simulink model "Desc_model"  (R2017a)
settings: Solver=VariableStepAuto  StartTime=0.0  StopTime=9.9  RelTol=1e-3
values from neighbouring files (symbols this model uses):
  A = double(subs(A_sym, phi_sym, 0))    [create_constants.m]    (also in forward_kinematic_linear.m = [0.7689, 0.0639, -0.1471, 0.0592; linearize_model.m = -1*((Rt / k_m * Z)\(Rt / k_m * V + EM * eye(4,4))); sim_system.m; test.m = [cos(phi), -sin(phi), 0)
  B = double(subs(B_sym, phi_sym, 0))    [create_constants.m]    (also in forward_kinematic_linear.m = [6.8984, -1.9066, 4.3907, -1.7678; linearize_model.m = pinv(Rt / k_m * Z); sim_system.m; test.m = [m, 0, 0)
  BotToWheel = G' / r    [create_constants.m]    (also in find_body_to_wheel_alpha.m = (-1 * G / r)'; graph_max_robot_speeds.m; sim_system.m; test_kalman_filter_LQI.m = -1 * G' / r)
  C = eye(4,4)    [create_constants.m]    (also in sim_system.m; test.m = simplify(C); test_kalman_filter_LQI.m; test_kalman_filter_LQR.m)
  camera_ts = 0.01    [create_constants.m]
  D = zeros(4,4)    [create_constants.m]    (also in sim_system.m; test.m = pinv(G); test_kalman_filter_LQI.m; test_kalman_filter_LQR.m)
  delay_sample = 0    [create_constants.m]
  encoder_ts = 0.01    [create_constants.m]
  td = 0    [create_constants.m]    (also in sim_system.m)
  ti = 0    [create_constants.m]    (also in sim_system.m)
  tp = 0    [create_constants.m]    (also in sim_system.m = 2)
  wd = 0    [create_constants.m]    (also in sim_system.m)
  WheelToBot = pinv(BotToWheel)    [create_constants.m]    (also in graph_max_robot_speeds.m; sim_system.m; test_kalman_filter_LQI.m; test_kalman_filter_LQR.m)
  wi = 0    [create_constants.m]    (also in sim_system.m = 0.5)
  wp = 0    [create_constants.m]    (also in sim_system.m = 1)
  X_0 = [0, 0, 0, 0]    [create_constants.m]
undefined symbols (not defined in the file or in its folder): K_int
libraries: simulink x4
settings Model: Creator=Joe  LastModifiedBy=Joe

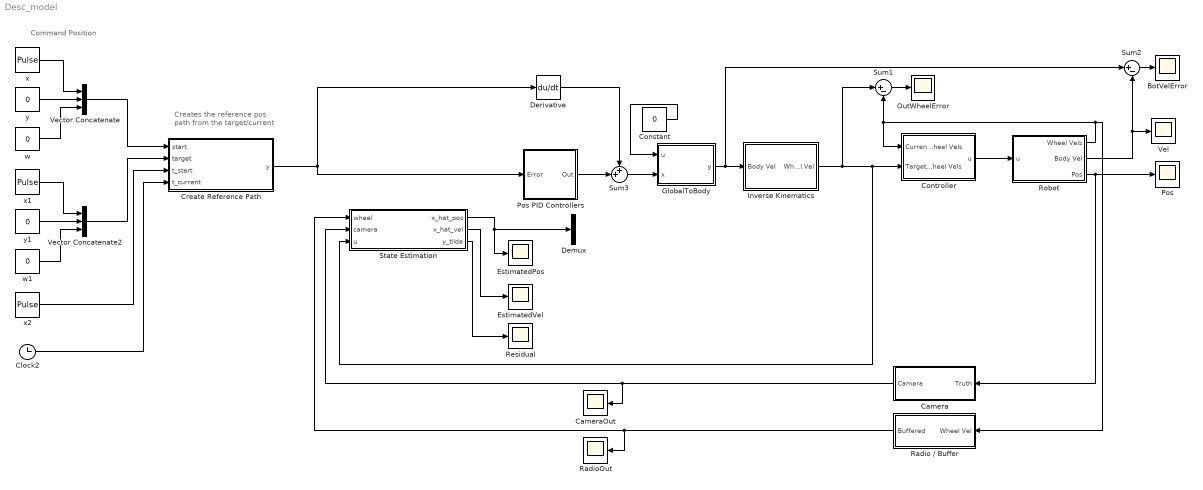
== system Desc_model ==
  note: Command Position
  note: Creates the reference pos
      | path from the target/current
  BotVelError : Scope
  Camera : Subsystem
  CameraOut : Scope
  Clock2 : Clock
  Constant : Constant  Value=0
  Controller : Subsystem
  Create Reference Path : MATLAB Function  TreatAsAtomicUnit=on
  Demux : Demux  Outputs=3
  Derivative : Derivative
  EstimatedPos : Scope
  EstimatedVel : Scope
  GlobalToBody : MATLAB Function  TreatAsAtomicUnit=on
  Inverse Kinematics : Subsystem
  OutWheelError : Scope
  Pos : Scope
  Pos PID Controllers : Subsystem
  Radio / Buffer : Subsystem
  RadioOut : Scope
  Residual : Scope
  Robot : Subsystem
  State Estimation : MATLAB Function  TreatAsAtomicUnit=on
  Sum1 : Sum  Inputs=|+-
  Sum2 : Sum  Inputs=|+-
  Sum3 : Sum  Inputs=++|
  Vector Concatenate : Concatenate  NumInputs=3
  Vector Concatenate2 : Concatenate  NumInputs=3
  Vel : Scope
  w : Constant  Value=0
  w1 : Constant  Value=0
  x : DiscretePulseGenerator  PulseType=Time based  Period=10  PulseWidth=50  PhaseDelay=5
  x1 : DiscretePulseGenerator  PulseType=Time based  Period=10  PulseWidth=50
  x2 : DiscretePulseGenerator  PulseType=Time based  Amplitude=5  Period=20  PulseWidth=50  PhaseDelay=5
  y : Constant  Value=0
  y1 : Constant  Value=0
  wires:
  Sum1/1 -> OutWheelError/1
  Sum2/1 -> BotVelError/1
  GlobalToBody/1(y) -> Sum2/1, Inverse Kinematics/1(Body Vel)
  Robot/1(Wheel Vels) -> Radio / Buffer/1(Wheel Vel), Controller/1(Current Wheel Vels), Sum1/2
  Controller/1(u) -> Robot/1(u)
  Inverse Kinematics/1(Wheel Vel) -> State Estimation/3(u), Controller/2(Target Wheel Vels), Sum1/1
  Robot/2(Body Vel) -> Vel/1, Sum2/2
  Robot/3(Pos) -> Camera/1(Truth), Pos/1
  w/1 -> Vector Concatenate/3
  Clock2/1 -> Create Reference Path/4(t_current)
  y/1 -> Vector Concatenate/2
  x1/1 -> Vector Concatenate2/1
  y1/1 -> Vector Concatenate2/2
  w1/1 -> Vector Concatenate2/3
  Vector Concatenate2/1 -> Create Reference Path/2(target)
  Vector Concatenate/1 -> Create Reference Path/1(start)
  x/1 -> Vector Concatenate/1
  x2/1 -> Create Reference Path/3(t_start)
  Camera/1(Camera) -> CameraOut/1, State Estimation/2(camera)
  Radio / Buffer/1(Buffered) -> RadioOut/1, State Estimation/1(wheel)
  State Estimation/1(x_hat_pos) -> Demux/1, EstimatedPos/1
  Sum3/1 -> GlobalToBody/2(x)
  Derivative/1 -> Sum3/1
  Pos PID Controllers/1(Out) -> Sum3/2
  State Estimation/3(y_tilda) -> Residual/1
  State Estimation/2(x_hat_vel) -> EstimatedVel/1
  Create Reference Path/1(y) -> Pos PID Controllers/1(Error), Derivative/1
  Constant/1 -> GlobalToBody/1(u)

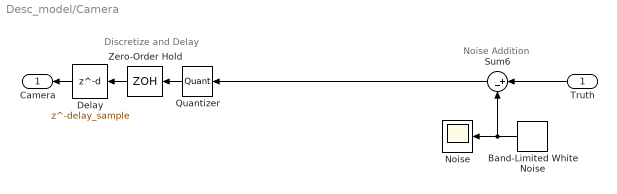
== system Desc_model/Camera ==
  note: Noise Addition
  note: Discretize and Delay
  Truth : Inport
  Band-Limited White Noise : simulink/Sources/Band-Limited White Noise  Cov=camera_noise  Ts=camera_ts  seed=[23341]
  Delay : Delay  DelayLength=delay_sample
  Noise : Scope
  Quantizer : Quantizer  QuantizationInterval=0.01
  Sum6 : Sum  Inputs=|+-
  Zero-Order Hold : ZeroOrderHold  SampleTime=camera_ts
  Camera : Outport
  wires:
  Delay/1 -> Camera/1
  Truth/1 -> Sum6/1
  Band-Limited White Noise/1 -> Noise/1, Sum6/2
  Quantizer/1 -> Zero-Order Hold/1
  Zero-Order Hold/1 -> Delay/1
  Sum6/1 -> Quantizer/1

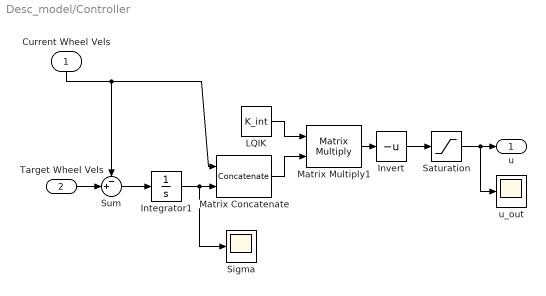
== system Desc_model/Controller ==
  Current Wheel Vels : Inport
  Target Wheel Vels : Inport  Port=2
  Integrator1 : Integrator
  Invert : UnaryMinus
  LQIK : Constant  Value=K_int
  Matrix Concatenate : Concatenate
  Matrix Multiply1 : Product  Multiplication=Matrix(*)
  Saturation : Saturate  UpperLimit=12  LowerLimit=-12
  Sigma : Scope
  Sum : Sum  Inputs=-+|
  u_out : Scope
  u : Outport
  wires:
  Invert/1 -> Saturation/1
  Integrator1/1 -> Sigma/1, Matrix Concatenate/2
  Sum/1 -> Integrator1/1
  Matrix Multiply1/1 -> Invert/1
  LQIK/1 -> Matrix Multiply1/1
  Matrix Concatenate/1 -> Matrix Multiply1/2
  Current Wheel Vels/1 -> Matrix Concatenate/1, Sum/1
  Target Wheel Vels/1 -> Sum/2
  Saturation/1 -> u_out/1, u/1

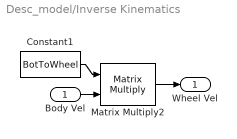
== system Desc_model/Inverse Kinematics ==
  Body Vel : Inport
  Constant1 : Constant  Value=BotToWheel
  Matrix Multiply2 : Product  Multiplication=Matrix(*)
  Wheel Vel : Outport
  wires:
  Constant1/1 -> Matrix Multiply2/1
  Body Vel/1 -> Matrix Multiply2/2
  Matrix Multiply2/1 -> Wheel Vel/1

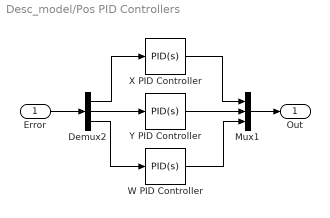
== system Desc_model/Pos PID Controllers ==
  Error : Inport
  Demux2 : Demux  Outputs=3
  Mux1 : Mux  Inputs=3
  W PID Controller : simulink/Continuous/PID Controller  Controller=PID  TimeDomain=Continuous-time  SampleTime=-1  IntegratorMethod=Forward Euler  FilterMethod=Forward Euler  Form=Parallel  UseFilter=on  ControllerParametersSource=internal  P=wp  I=wi  D=wd  N=26080.4758865559  InitialConditionSource=internal  InitialConditionForIntegrator=0  InitialConditionForFilter=0  ExternalReset=none  LimitOutput=off  UpperSaturationLimit=inf  LowerSaturationLimit=-inf  LinearizeAsGain=on  AntiWindupMode=none  Kb=1  TrackingMode=off  Kt=1  PParamMin=[]  PParamMax=[]  IParamMin=[]  IParamMax=[]  DParamMin=[]  DParamMax=[]  NParamMin=[]  NParamMax=[]  KbParamMin=[]  KbParamMax=[]  KtParamMin=[]  KtParamMax=[]  POutMin=[]  POutMax=[]  IOutMin=[]  IOutMax=[]  DOutMin=[]  DOutMax=[]  NOutMin=[]  NOutMax=[]  KbOutMin=[]  KbOutMax=[]  KtOutMin=[]  KtOutMax=[]  IntegratorOutMin=[]  IntegratorOutMax=[]  FilterOutMin=[]  FilterOutMax=[]  SumOutMin=[]  SumOutMax=[]  SumI1OutMin=[]  SumI1OutMax=[]  SumI2OutMin=[]  SumI2OutMax=[]  SumI3OutMin=[]  SumI3OutMax=[]  SumDOutMin=[]  SumDOutMax=[]  SaturationOutMin=[]  SaturationOutMax=[]  IntegratorContinuousStateAttributes=''  IntegratorStateMustResolveToSignalObject=off  IntegratorRTWStateStorageClass=Auto  FilterContinuousStateAttributes=''  FilterStateMustResolveToSignalObject=off  FilterRTWStateStorageClass=Auto  DifferentiatorICPrevScaledInput=0  DifferentiatorOutMin=[]  DifferentiatorOutMax=[]  InitialConditionSetting=State (most efficient)
  X PID Controller : simulink/Continuous/PID Controller  Controller=PID  TimeDomain=Continuous-time  SampleTime=-1  IntegratorMethod=Forward Euler  FilterMethod=Forward Euler  Form=Parallel  UseFilter=on  ControllerParametersSource=internal  P=tp  I=ti  D=td  N=0  InitialConditionSource=internal  InitialConditionForIntegrator=0  InitialConditionForFilter=0  ExternalReset=none  LimitOutput=off  UpperSaturationLimit=inf  LowerSaturationLimit=-inf  LinearizeAsGain=on  AntiWindupMode=none  Kb=1  TrackingMode=off  Kt=1  PParamMin=[]  PParamMax=[]  IParamMin=[]  IParamMax=[]  DParamMin=[]  DParamMax=[]  NParamMin=[]  NParamMax=[]  KbParamMin=[]  KbParamMax=[]  KtParamMin=[]  KtParamMax=[]  POutMin=[]  POutMax=[]  IOutMin=[]  IOutMax=[]  DOutMin=[]  DOutMax=[]  NOutMin=[]  NOutMax=[]  KbOutMin=[]  KbOutMax=[]  KtOutMin=[]  KtOutMax=[]  IntegratorOutMin=[]  IntegratorOutMax=[]  FilterOutMin=[]  FilterOutMax=[]  SumOutMin=[]  SumOutMax=[]  SumI1OutMin=[]  SumI1OutMax=[]  SumI2OutMin=[]  SumI2OutMax=[]  SumI3OutMin=[]  SumI3OutMax=[]  SumDOutMin=[]  SumDOutMax=[]  SaturationOutMin=[]  SaturationOutMax=[]  IntegratorContinuousStateAttributes=''  IntegratorStateMustResolveToSignalObject=off  IntegratorRTWStateStorageClass=Auto  FilterContinuousStateAttributes=''  FilterStateMustResolveToSignalObject=off  FilterRTWStateStorageClass=Auto  DifferentiatorICPrevScaledInput=0  DifferentiatorOutMin=[]  DifferentiatorOutMax=[]  InitialConditionSetting=State (most efficient)
  Y PID Controller : simulink/Continuous/PID Controller  Controller=PID  TimeDomain=Continuous-time  SampleTime=-1  IntegratorMethod=Forward Euler  FilterMethod=Forward Euler  Form=Parallel  UseFilter=on  ControllerParametersSource=internal  P=tp  I=ti  D=td  N=0  InitialConditionSource=internal  InitialConditionForIntegrator=0  InitialConditionForFilter=0  ExternalReset=none  LimitOutput=off  UpperSaturationLimit=inf  LowerSaturationLimit=-inf  LinearizeAsGain=on  AntiWindupMode=none  Kb=1  TrackingMode=off  Kt=1  PParamMin=[]  PParamMax=[]  IParamMin=[]  IParamMax=[]  DParamMin=[]  DParamMax=[]  NParamMin=[]  NParamMax=[]  KbParamMin=[]  KbParamMax=[]  KtParamMin=[]  KtParamMax=[]  POutMin=[]  POutMax=[]  IOutMin=[]  IOutMax=[]  DOutMin=[]  DOutMax=[]  NOutMin=[]  NOutMax=[]  KbOutMin=[]  KbOutMax=[]  KtOutMin=[]  KtOutMax=[]  IntegratorOutMin=[]  IntegratorOutMax=[]  FilterOutMin=[]  FilterOutMax=[]  SumOutMin=[]  SumOutMax=[]  SumI1OutMin=[]  SumI1OutMax=[]  SumI2OutMin=[]  SumI2OutMax=[]  SumI3OutMin=[]  SumI3OutMax=[]  SumDOutMin=[]  SumDOutMax=[]  SaturationOutMin=[]  SaturationOutMax=[]  IntegratorContinuousStateAttributes=''  IntegratorStateMustResolveToSignalObject=off  IntegratorRTWStateStorageClass=Auto  FilterContinuousStateAttributes=''  FilterStateMustResolveToSignalObject=off  FilterRTWStateStorageClass=Auto  DifferentiatorICPrevScaledInput=0  DifferentiatorOutMin=[]  DifferentiatorOutMax=[]  InitialConditionSetting=State (most efficient)
  Out : Outport
  wires:
  Error/1 -> Demux2/1
  Mux1/1 -> Out/1
  X PID Controller/1 -> Mux1/1
  Demux2/2 -> Y PID Controller/1
  W PID Controller/1 -> Mux1/3
  Demux2/1 -> X PID Controller/1
  Y PID Controller/1 -> Mux1/2
  Demux2/3 -> W PID Controller/1

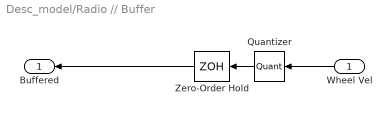
== system Desc_model/Radio // Buffer ==
  Wheel Vel : Inport
  Quantizer : Quantizer  QuantizationInterval=0.01
  Zero-Order Hold : ZeroOrderHold  SampleTime=encoder_ts
  Buffered : Outport
  wires:
  Zero-Order Hold/1 -> Buffered/1
  Wheel Vel/1 -> Quantizer/1
  Quantizer/1 -> Zero-Order Hold/1

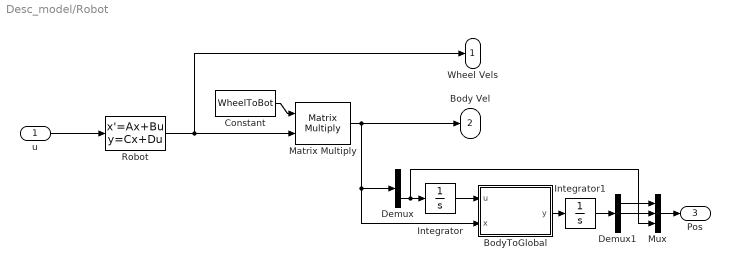
== system Desc_model/Robot ==
  u : Inport
  BodyToGlobal : MATLAB Function  TreatAsAtomicUnit=on
  Constant : Constant  Value=WheelToBot
  Demux : Demux  Outputs=3
  Demux1 : Demux  Outputs=3
  Integrator : Integrator
  Integrator1 : Integrator
  Matrix Multiply : Product  Multiplication=Matrix(*)
  Mux : Mux  Inputs=3
  Robot : StateSpace  A=A  B=B  C=C  D=D  X0=X_0
  Wheel Vels : Outport
  Body Vel : Outport  Port=2
  Pos : Outport  Port=3
  wires:
  Robot/1 -> Wheel Vels/1, Matrix Multiply/2
  Matrix Multiply/1 -> BodyToGlobal/2(x), Demux/1, Body Vel/1
  Constant/1 -> Matrix Multiply/1
  u/1 -> Robot/1
  Demux/3 -> Mux/3, Integrator/1
  Integrator/1 -> BodyToGlobal/1(u)
  Demux1/2 -> Mux/2
  Demux1/1 -> Mux/1
  Mux/1 -> Pos/1
  BodyToGlobal/1(y) -> Integrator1/1
  Integrator1/1 -> Demux1/1

== matlab function Desc_model/Create Reference Path ==
  data: start input; target input; y output; t_start input; t_current input
function y = Create_Ref(start, target, t_start, t_current)
y = zeros(3,1);
for i = 1:3
    a_c = 2; % Max Accel
    s_c = 1; % Max Speed
    t_a = s_c / a_c;
    
    sign = 2*(target(i) > start(i)) - 1;
    
    t_s = sign*(target(i) - start(i))/s_c - t_a;
    t_end = t_start + t_a + t_s + t_a;

    if (abs(start(i) - target(i)) < 0.01)
        y(i) = 0;
        continue;
    end
    
    if t_current < t_start
        y(i) = start(i);
    elseif t_current < t_start + t_a
        y(i) = start(i) + sign*1/2*a_c*(t_current - t_start)^2;
    elseif t_current < t_end - t_a
        y(i) = 1/2*(start(i) + target(i)) + sign*s_c*(t_current - 1/2*(t_start + t_end));
    elseif t_current < t_end
        y(i) = target(i) - sign*1/2*a_c*(t_end - t_current)^2;
    else % t_current > t_end
        y(i) = target(i);
    end
end

== matlab function Desc_model/Robot/BodyToGlobal ==
  data: u input; y output; x input
function y =  rotate(u, x)

r = [cos(u), -sin(u), 0;
     sin(u),  cos(u), 0;
          0,       0, 1];
y = r*x;

== matlab function Desc_model/GlobalToBody ==
  data: u input; y output; x input
function y =  rotate(u, x)

r = [cos(u), -sin(u), 0;
     sin(u),  cos(u), 0;
          0,       0, 1];
y = r*x;

== matlab function Desc_model/State Estimation ==
  data: wheel input; camera input; u input; x_hat_pos output; x_hat_vel output; y_tilda output
function [x_hat_pos, x_hat_vel, y_tilda] = state_estimation(wheel, camera, u)
% Camera defaults to 0
% when we get a new camera value, reset kalman filter and recalcultate
persistent previous_wheel;
persistent camera_x_hat_k1_k1;
persistent camera_P_k1_k1;
persistent x_hat_k1_k1;
persistent P_k1_k1;

% global F_k; % A
% global B_k; % B
% global H_k; % C
% global Q_k; % Covariance of process noise
% global R_k; % Covariance of observation noise
% global I;

coder.extrinsic('evalin');
F_k = zeros(15,15);
B_k = zeros(15,15);
H_k = zeros(7,15);
Q_k = zeros(15,15);
R_k = zeros(7,7);
I = eye(15,15);
F_k = evalin('base', 'F_k');
B_k = evalin('base', 'B_k');
H_k = evalin('base', 'H_k');
Q_k = evalin('base', 'Q_k');
R_k = evalin('base', 'R_k');

delay_sample = 0;
delay_sample = evalin('base', 'delay_sample');

if isempty(x_hat_k1_k1)
    x_hat_k1_k1 = zeros(15,1);
end

if isempty(P_k1_k1)
    P_k1_k1 = zeros(15, 15);
end

if isempty(previous_wheel)
    if delay_sample ~= 0
        previous_wheel = zeros(4, delay_sample);
    else
        previous_wheel = [];
    end
end

if isempty(camera_x_hat_k1_k1)
    camera_x_hat_k1_k1 = zeros(15, 1);
end

if isempty(camera_P_k1_k1)
    camera_P_k1_k1 = zeros(15, 15);
end

if (delay_sample ~= 0)
    previous_wheel = [previous_wheel, wheel];
    
    % Reset to old camera x_hat_k1_k1 and P_k1_k1
    % Eval once and save to camera x_hat_k1_k1 and P_k1_k1
    % Loop for each wheel update
end

% Output data from plant
z_k = [camera; wheel];
u = [0;0;0;u;0;0;0;0;0;0;0;0];
% Predict where we should be this time step
x_hat_k_k1 = F_k*x_hat_k1_k1 + B_k*u;
P_k_k1 = F_k*P_k1_k1*F_k' + Q_k;

% Get error between predicted and actual
y_tilda_k = z_k - H_k*x_hat_k_k1;
S_k = R_k + H_k*P_k_k1*H_k';

% Get optimal state estimator gain
K_k = P_k_k1*H_k'*pinv(S_k);

% Update state
x_hat_k_k = x_hat_k_k1 + K_k*y_tilda_k;

% Update final covariance / better output
P_k_k = (I - K_k*H_k)*P_k_k1*(I - K_k*H_k)' + K_k*R_k*K_k';
y_tilda_k_k = z_k - H_k*x_hat_k_k;

x_hat_pos = x_hat_k_k(1:3);
x_hat_vel = x_hat_k_k(4:8);
y_tilda = y_tilda_k_k;

% Setup P for the next iteration
P_k1_k1 = P_k_k;
x_hat_k1_k1 = x_hat_k_k;
end
